simulink model "simulacionaudio"  (R2018a)
settings: Solver=VariableStepAuto  StartTime=0.0  StopTime=4  RelTol=1e-3
libraries: dsparch4 x2, commutil2 x2, dspsigops x2, dspquant2 x2, dspvision x1
settings Model: Creator=jario  LastModifiedBy=jario

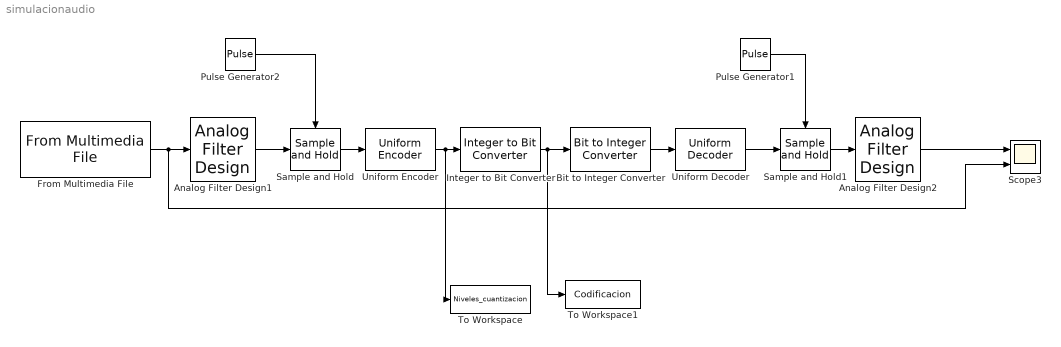
== system simulacionaudio ==
  Analog Filter Design1 : dsparch4/Analog Filter Design  method=Butterworth  filttype=Lowpass  N=10  Wlo=3400  Whi=4000  Rp=2  Rs=40
  Analog Filter Design2 : dsparch4/Analog Filter Design  method=Butterworth  filttype=Lowpass  N=10  Wlo=3400  Whi=4000  Rp=2  Rs=40
  Bit to Integer Converter : commutil2/Bit to Integer Converter  nbits=32  bitOrder=MSB first  signedOutputValues=Signed  outDtype=Inherit via internal rule  outDtypeSigned=Inherit via internal rule
  From Multimedia File : dspvision/From Multimedia File  inputFilename=C:\Users\jario\Documents\Universidad de Medellin\Señales y Sistemas ll\SenSis2_Cod3\SenSis2_Cod3\audiograbado.wav  loop=on  numPlays=inf  outputStreams=Audio only  videoDataType=single  audioDataType=double  inheritSampleTime=off  userDefinedSampleTime=1/8000  noAudioOutput=off  isIntensityVideo=off  fourcc=RGB  colorVideoFormat=Separate color signals  outputEOF=off  dataOrg=Column-major  audioFrameSize=1  computeAudioFrameSize=off  outSamplingMode=Sample based
      settings: SourceProductBaseCode=VP
  Integer to Bit Converter : commutil2/Integer to Bit Converter  nbits=32  signedInputValues=Signed  bitOrder=MSB first  outDtype=Inherit via internal rule
  Pulse Generator1 : DiscretePulseGenerator  PulseType=Time based  Period=1/8000  PulseWidth=50
  Pulse Generator2 : DiscretePulseGenerator  PulseType=Time based  Period=1/8000  PulseWidth=50
  Sample and Hold : dspsigops/Sample and Hold  trig=Rising edge  initCond=0  latchinput=off
  Sample and Hold1 : dspsigops/Sample and Hold  trig=Rising edge  initCond=0  latchinput=off
  Scope3 : Scope  NumInputPorts=2
  To Workspace : ToWorkspace  VariableName=Niveles_cuantizacion  SampleTime=-1
      settings: Save2DSignal=2-D array (concatenate along first dimension)
  To Workspace1 : ToWorkspace  VariableName=Codificacion  SampleTime=-1
      settings: Save2DSignal=2-D array (concatenate along first dimension)
  Uniform Decoder : dspquant2/Uniform Decoder  peak=1  bits=32  overflowMode=Saturate  otype=Double
      settings: SourceProductName=DSP System Toolbox  SourceProductBaseCode=DS
  Uniform Encoder : dspquant2/Uniform Encoder  peak=1  bits=32  otype=Signed integer
      settings: SourceProductName=DSP System Toolbox
  wires:
  Pulse Generator2/1 -> Sample and Hold/Trigger
  Integer to Bit Converter/1 -> To Workspace1/1, Bit to Integer Converter/1
  Pulse Generator1/1 -> Sample and Hold1/Trigger
  Bit to Integer Converter/1 -> Uniform Decoder/1
  Uniform Decoder/1 -> Sample and Hold1/1
  Sample and Hold/1 -> Uniform Encoder/1
  Uniform Encoder/1 -> To Workspace/1, Integer to Bit Converter/1
  Sample and Hold1/1 -> Analog Filter Design2/1
  Analog Filter Design1/1 -> Sample and Hold/1
  From Multimedia File/1 -> Scope3/2, Analog Filter Design1/1
  Analog Filter Design2/1 -> Scope3/1
